simulink model "LAB2_2"  (R2017b)
settings: Solver=VariableStepAuto  StartTime=0.0  StopTime=10.0  RelTol=1e-3
libraries: simulink x1
settings Model: Creator=ArsalanBangash  LastModifiedBy=ArsalanBangash

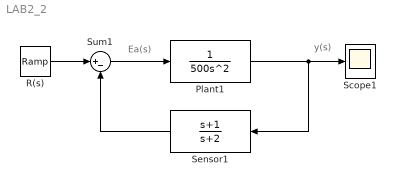
== system LAB2_2 ==
  note: Ea(s)
  note: y(s)
  Plant1 : TransferFcn  Denominator=[500 0 0]
  R(s) : simulink/Sources/Ramp  slope=2  start=0  X0=0
  Scope1 : Scope
  Sensor1 : TransferFcn  Numerator=[1 1]  Denominator=[1 2]
  Sum1 : Sum  Inputs=|+-
  wires:
  Sensor1/1 -> Sum1/2
  R(s)/1 -> Sum1/1
  Sum1/1 -> Plant1/1
  Plant1/1 -> Scope1/1, Sensor1/1
